simulink model "straightRoadVideoRecording"  (R2022a)
settings: Solver=VariableStepAuto  StartTime=0.0  StopTime=1  RelTol=1e-3
libraries: sim3dcameralib x2, sim3dlib x1, sim3dautolib x1
settings Model: Creator=The MathWorks, Inc.  LastModifiedBy=Administrator
settings SolverCC: AlgebraicLoopSolver=TrustRegion
settings DebuggingCC: UnconnectedInputMsg=warning  UnconnectedOutputMsg=warning  UnconnectedLineMsg=warning  SFMachineParentedDataDiag=warning
settings RTWCC: DLArmComputeVersion=19.05

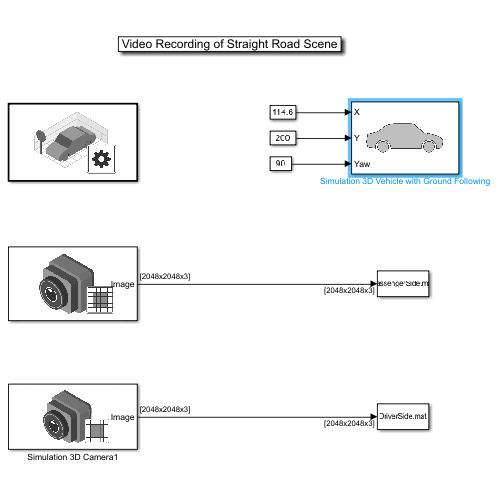
[thumbnail: Simulink's stored preview of the top-level diagram]
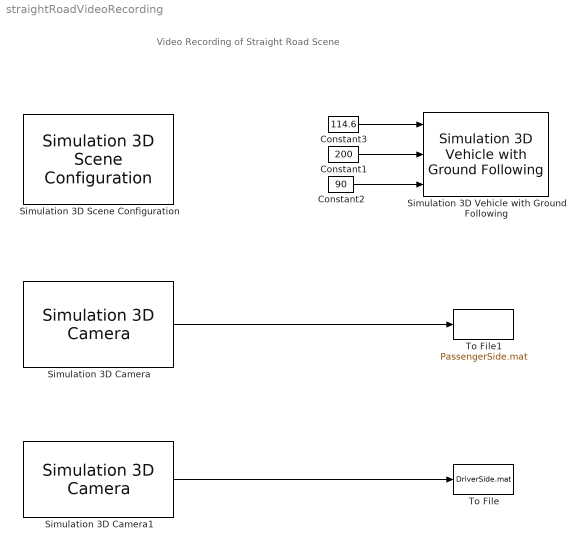
== system straightRoadVideoRecording ==
  note: Video Recording of Straight Road Scene
  Constant1 : Constant  Value=200
  Constant2 : Constant  Value=90
  Constant3 : Constant  Value=114.6
  Simulation 3D Camera : sim3dcameralib/Simulation 3D Camera  Priority=1  sensorTag=Sim3dSensor4  sensorId=4  sensorName=Sim3dSensor4  vehTagList={'Scene Origin';'SimulinkVehicle1'}  vehTag=SimulinkVehicle1  mountLoc=Origin  offsetFlag=on  tmountOffset=CameraPosiP  extTmount=off  rmountOffset=CameraAngsP  extRmount=off  FocalLength=CameraF_P  OpticalCenter=CameraOPCenterP  ImageSize=imagesizeP  RadialDistortion=[0, 0]  TangentialDistortion=[0, 0]  SensorSkew=0  DepthOutportEnabled=off  SemanticOutportEnabled=off  TransformOutportEnabled=off  SampleTime=-1  mountPoint=[0.237263 1.11436 1.10793]  mountOrientation=[180 -176.29 -16.96]  aMode=3  ID=4
      settings: SourceProductBaseCode=VE,AE,DR,UV,VE
  Simulation 3D Camera1 : sim3dcameralib/Simulation 3D Camera  sensorTag=Sim3dSensor3  sensorId=3  sensorName=Sim3dSensor3  vehTagList={'Scene Origin';'SimulinkVehicle1'}  vehTag=SimulinkVehicle1  mountLoc=Origin  offsetFlag=on  tmountOffset=CameraPosi  extTmount=off  rmountOffset=CameraAngs  extRmount=off  FocalLength=CameraF  OpticalCenter=CameraOPCenter  ImageSize=imagesize  RadialDistortion=[0, 0]  TangentialDistortion=[0, 0]  SensorSkew=0  DepthOutportEnabled=off  SemanticOutportEnabled=off  TransformOutportEnabled=off  SampleTime=-1  mountPoint=[0.237263 -1.11436 1.10793]  mountOrientation=[180 -176.29 16.96]  aMode=3  ID=3
      settings: SourceProductBaseCode=VE,AE,DR,UV,VE
  Simulation 3D Scene Configuration : sim3dlib/Simulation 3D Scene Configuration  Priority=0  ProjectFormat=Default Scenes  SceneDesc=Virtual Mcity  ProjectName=C:\Program Files\MATLAB\R2022a\toolbox\shared\sim3d_projects\automotive_project\UE4\WindowsNoEditor\VehicleSimulation.exe  ScenePath=/Game/Maps/HwStrght  vehTagList={'Scene Origin';'SimulinkVehicle1'}  vehTag=SimulinkVehicle1  OpVisEn=off  Ts=1  EnableWindow=on  EnableRemoteAccess=off  EnableWeather=on  SunAltitude=90.0  SunAzimuth=187.200  clouds=10  wind=1  fog=0  rain=0  sensorTag=MainCamera2  sensorId=2  sensorName=MainCamera2  mountLoc=Origin  offsetFlag=off  tmountOffset=[0, 0, 0]  rmountOffset=[0, 0, 0]  HorizontalResolution=1280  VerticalResolution=720  HorizontalFOV=60  mountPoint=[0 0 0]  mountOrientation=[0 0 0]  aMode=3  ID=2
      settings: SourceProductBaseCode=VE,AE,DR,UV,VE
  Simulation 3D Vehicle with Ground Following : sim3dautolib/Simulation 3D Vehicle with Ground Following  Priority=-1  PassVehMesh=Small pickup truck  MeshPath=/MathWorksSimulation/Vehicles/Muscle/Meshes/SK_MuscleCar.SK_MuscleCar  TrackWidth=1.9  WheelBase=3  WheelRadius=0.35  VehColor=Silver  InitialPos=[0, 0, 0]  InitialRot=[0, 0, 0]  ActorName=SimulinkVehicle1  SampleTime=-1  ActorType=SimulinkVehicle  ID=1  aMode=3  ActorTag=SimulinkVehicle1  CoordinateScheme=ISO  VehLightsControl=off  HeadlightColor=[ 1, 1, 1 ]  HighBeamIntensity=100000  LowBeamIntensity=60000  HighBeamConeAngle=70  LowBeamConeAngle=70  LeftHeadlightOrientation=[ 0, 0 ]  RightHeadlightOrientation=[ 0, 0 ]  BrakelightIntensity=500  ReverselightIntensity=500  SignallightIntensity=500  SignallightPeriod=1  SignalPulseWidth=50  TransformOutportEnabled=off
      settings: SourceProductBaseCode=VE,AE,DR,UV,VE
  To File : ToFile  Filename=DriverSide.mat  SaveFormat=Timeseries
  To File1 : ToFile  Filename=PassengerSide.mat  SaveFormat=Timeseries
  wires:
  Constant1/1 -> Simulation 3D Vehicle with Ground Following/2
  Constant2/1 -> Simulation 3D Vehicle with Ground Following/3
  Simulation 3D Camera1/1 -> To File/1
  Simulation 3D Camera/1 -> To File1/1
  Constant3/1 -> Simulation 3D Vehicle with Ground Following/1
